simulink model "HighpassFilter"  (R2020a)
settings: Solver=VariableStepAuto  StartTime=0.0  StopTime=10.0  RelTol=1e-3
libraries: dspfdesign x1
settings Model: Creator=Hp  LastModifiedBy=Hp

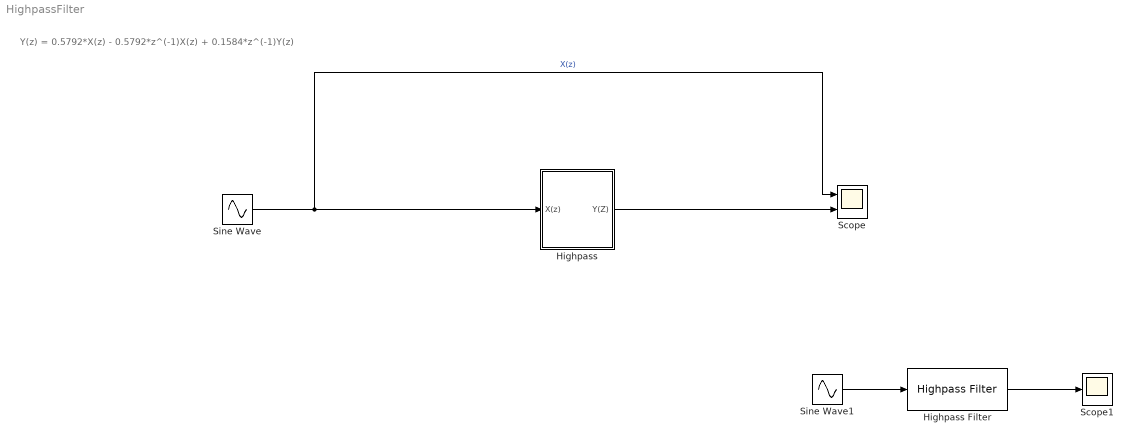
== system HighpassFilter ==
  note: Y(z) = 0.5792*X(z) - 0.5792*z^(-1)X(z) + 0.1584*z^(-1)Y(z)
  Highpass : Subsystem
  Highpass Filter : dspfdesign/Highpass Filter  FilterType=FIR  DesignForMinimumOrder=on  FilterOrder=50  StopbandFrequency=8e3  PassbandFrequency=12e3  StopbandAttenuation=80  PassbandRipple=0.1  InheritSampleRate=off  SampleRate=44100  SimulateUsing=Interpreted execution  roundingMode=Floor  coeffsDataTypeStr=fixdt(1,16)
  Scope : Scope  NumInputPorts=2
  Scope1 : Scope
  Sine Wave : Sin  Frequency=2*pi*7000  SampleTime=1/5000
  Sine Wave1 : Sin  Frequency=2*pi*7000  SampleTime=1/5000
  wires:
  Sine Wave/1 -> Scope/1, Highpass/1(X(z))  "X(z)"
  Highpass/1(Y(Z)) -> Scope/2
  Sine Wave1/1 -> Highpass Filter/1
  Highpass Filter/1 -> Scope1/1

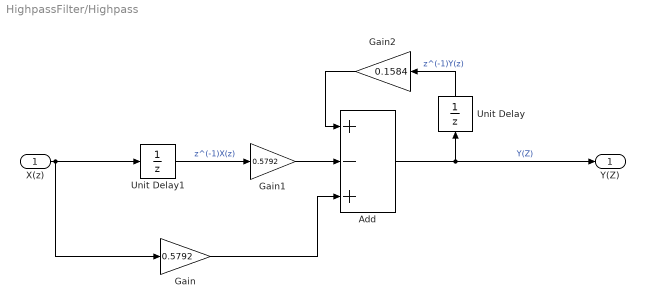
== system HighpassFilter/Highpass ==
  X(z) : Inport
  Add : Sum  Inputs=+-+
  Gain : Gain  Gain=0.5792
  Gain1 : Gain  Gain=0.5792
  Gain2 : Gain  Gain=0.1584
  Unit Delay : UnitDelay  SampleTime=-1  HasFrameUpgradeWarning=on
  Unit Delay1 : UnitDelay  SampleTime=-1  HasFrameUpgradeWarning=on
  Y(Z) : Outport
  wires:
  Add/1 -> Y(Z)/1, Unit Delay/1  "Y(Z)"
  Gain/1 -> Add/3
  Gain1/1 -> Add/2
  Gain2/1 -> Add/1
  Unit Delay1/1 -> Gain1/1  "z^(-1)X(z)"
  X(z)/1 -> Gain/1, Unit Delay1/1
  Unit Delay/1 -> Gain2/1  "z^(-1)Y(z)"
